simulink library "thc"  (R2021b)
settings: Solver=VariableStepAuto  StartTime=0.0  StopTime=10.0  RelTol=1e-3
undefined symbols (not defined in the file or in its folder): ATHC_APTCQA_X_C, ATHC_APTCQB_X_C, ATHC_dAy_X_C, ATHC_Qeq_X_kmh, ATHC_VbaseC_X_C, ATHC_VbaseC_Y_W, ATHC_VbaseD_X_C, ATHC_VbaseH_X_C, FALSE, KTHC_ACMaxMinT_sec, KTHC_aDeice_K, KTHC_AGSDefLv_K, KTHC_AGSLv1_K, KTHC_AGSLv2_K, KTHC_AGSLv3_K, KTHC_AGSLv4_K, KTHC_AGSLv5_K, KTHC_AirIntUpdateT_sec, KTHC_APTCOneZoneMax_W, KTHC_APTCPeriod_cnt, KTHC_APTCPWMEN_flg, KTHC_APTCQMaxC_W, KTHC_APTCQminC_W, KTHC_APTCQminD_W, KTHC_APTCQminRe1_W, KTHC_APTCQminRe_W, KTHC_APTCQoffT_cnt, KTHC_APTCQonT_cnt, KTHC_APTCRiLeMaxDff_W, KTHC_APTCRiLeMinDff_W, KTHC_BatInTempDef_C, KTHC_bDeice_K, KTHC_CompMaxDeice_rpm, KTHC_CompMinDeice_rpm, KTHC_CompSotxvOp_K, KTHC_CompSotxvOpLow_rpm, KTHC_CompSpdmax_rpm, KTHC_CompSpdmaxBC1_rpm, KTHC_CompSpdmaxBC_rpm, KTHC_CompSpdmid1_rpm, KTHC_CompSpdmid2_rpm, KTHC_CompSpdmid3_rpm, KTHC_CompSpdmid_rpm, KTHC_CompSpdmin_rpm, KTHC_DAPTCQ1_W, KTHC_DAPTCQ2_W, KTHC_DAPTCQ3_W, KTHC_DcChSetTemp_C, KTHC_DehumidityEN_flg, KTHC_DeiceCycTime_K, KTHC_DriveLevelWPTCBAH1_W, KTHC_DriveLevelWPTCBAH2_W, KTHC_DriveLevelWPTCBAH3_W, KTHC_DriveLevelWPTCBAH4_W, KTHC_DriveT1MinBAH_C, KTHC_DriveT2MaxBAH_C, KTHC_DriveT2MinBAH_C, KTHC_DriveT3MaxBAH_C, KTHC_DriveT3MinBAH_C, KTHC_DriveT4MaxBAH_C ... (+377)
libraries: simulink x145
(part 5 of 10)

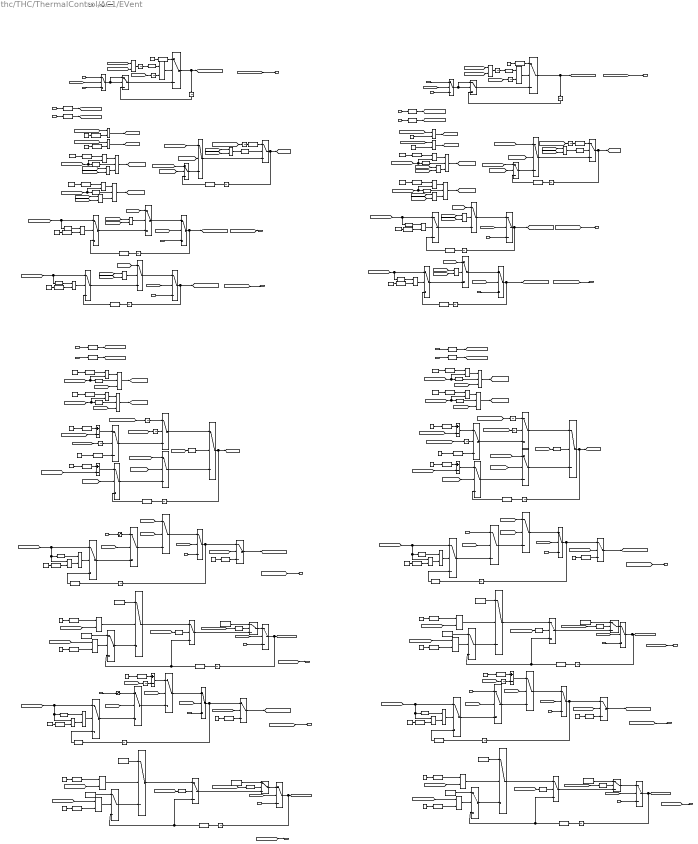
== system thc/THC/ThermalControl/AC1/EVent ==
  note: Driver Side
  note: Passenger Side
  fInitial : Inport
  VINP_IVIDrBlowerModeSta_enum : Inport  Port=2
  VINP_FDCTHCDrEVentModeStaM_enum : Inport  Port=3
  VINP_IVIPsBlowerModeSta_enum : Inport  Port=4
  VINP_FDCTHCPsEVentModeStaM_enum : Inport  Port=5
  VINP_IVIDrBlowerZSta_enum : Inport  Port=6
  VINP_IVICLBlowerZSta_enum : Inport  Port=7
  VINP_IVIPsBlowerZSta_enum : Inport  Port=8
  VINP_IVICRBlowerZSta_enum : Inport  Port=9
  VINP_FDCTHCDrEVentZStaM_enum : Inport  Port=10
  VINP_FDCTHCCLEVentZStaM_enum : Inport  Port=11
  VINP_FDCTHCPsEVentZStaM_enum : Inport  Port=12
  VINP_FDCTHCCREVentZStaM_enum : Inport  Port=13
  VINP_IVIDrBlowerYSta_enum : Inport  Port=14
  VINP_IVICLBlowerYSta_enum : Inport  Port=15
  VINP_ZFRTHCDrEVentActYSta_enum : Inport  Port=16
  VTHC_FDCTHCDrVentENM_flg : Inport  Port=17
  VINP_FDCTHCDrEVentYStaM_enum : Inport  Port=18
  VINP_ZFRTHCCLEVentActYSta_enum : Inport  Port=19
  VTHC_FDCTHCCLVentENM_flg : Inport  Port=20
  VINP_FDCTHCCLEVentYStaM_enum : Inport  Port=21
  VINP_IVIPsBlowerYSta_enum : Inport  Port=22
  VINP_IVICRBlowerYSta_enum : Inport  Port=23
  VINP_ZFRTHCPsEVentActYSta_enum : Inport  Port=24
  VTHC_FDCTHCPsVentENM_flg : Inport  Port=25
  VINP_FDCTHCPsEVentYStaM_enum : Inport  Port=26
  VINP_ZFRTHCCREVentActYSta_enum : Inport  Port=27
  VTHC_FDCTHCCRVentENM_flg : Inport  Port=28
  VINP_FDCTHCCREVentYStaM_enum : Inport  Port=29
  Add{,1..5} (6 alike) : Sum  Inputs=+-
  Constant{,1,4..5,7..8,10,14,18,23,25,28..29,33,38,40..42,45..46,48..51,53..54} (26 alike) : Constant  Value=100
  Constant11 : Constant  Value=3
  Constant12 : Constant  Value=50
  Constant{6,9,13,19,24,34,39,47} (8 alike) : Constant  Value=true
  Constant{15..16,20..21,30..31,35..36} (8 alike) : Constant  Value=126
  Constant{17,22,32,37} (4 alike) : Constant  Value=false
  Constant2 : Constant  Value=2
  Constant26 : Constant  Value=3
  Constant27 : Constant  Value=50
  Constant3 : Constant  Value=2
  Constant43 : Constant
  Constant44 : Constant
  Data Type Conversion{,1..20,22..25,27..35,37..40,42..65} (62 alike) : DataTypeConversion  OutDataTypeStr=uint8
  Data Type Conversion{21,26,36,41} (4 alike) : DataTypeConversion  OutDataTypeStr=boolean
  Detect Change{,1..17,19..20} (20 alike) : simulink/Logic and Bit Operations/Detect Change  vinit=0  OutDataTypeStr=boolean
  Detect Decrease : simulink/Logic and Bit Operations/Detect Decrease  vinit=0.0  OutDataTypeStr=boolean
  Detect Decrease1 : simulink/Logic and Bit Operations/Detect Decrease  vinit=0.0  OutDataTypeStr=boolean
  Detect Increase{,1..7} (8 alike) : simulink/Logic and Bit Operations/Detect Increase  vinit=0.0  OutDataTypeStr=boolean
  Logical Operator{,1..3,5..8} (8 alike) : Logic  Inputs=3  AllPortsSameDT=off  OutDataTypeStr=boolean
  Logical Operator{9..12,22..25} (8 alike) : Logic  AllPortsSameDT=off  OutDataTypeStr=boolean
  Logical Operator{4,13..21} (10 alike) : Logic  Operator=OR  AllPortsSameDT=off  OutDataTypeStr=boolean
  Relational Operator{,1,4..5,7..8,22..23} (8 alike) : RelationalOperator  OutDataTypeStr=boolean  RndMeth=Simplest
  Relational Operator{2,9..10,13,15..16,19,21,24..25,27..28} (12 alike) : RelationalOperator  Operator=<=  OutDataTypeStr=boolean  RndMeth=Simplest
  Relational Operator{3,6,11..12,14,17..18,20} (8 alike) : RelationalOperator  Operator===  OutDataTypeStr=boolean  RndMeth=Simplest
  Saturation : Saturate  UpperLimit=100  LowerLimit=0
  Saturation1 : Saturate  UpperLimit=100  LowerLimit=0
  Switch{,1..73} (74 alike) : Switch  Criteria=u2 > Threshold
  Unit Delay{,1..31} (32 alike) : UnitDelay  SampleTime=-1  HasFrameUpgradeWarning=on
  VTHC_FDCTHCDrEVentModeSta_enum : Outport
  VTHC_FDCTHCPsEVentModeSta_enum : Outport  Port=2
  VTHC_FDCTHCDrEVentZSta_enum : Outport  Port=3
  VTHC_FDCTHCCLEVentZSta_enum : Outport  Port=4
  VTHC_FDCTHCPsEVentZSta_enum : Outport  Port=5
  VTHC_FDCTHCCREVentZSta_enum : Outport  Port=6
  VTHC_FDCTHCDrEVentYSta_enum : Outport  Port=7
  VTHC_FDCTHCDrVentEN_flg : Outport  Port=8
  VTHC_FDCTHCCLEVentYSta_enum : Outport  Port=9
  VTHC_FDCTHCCLVentEN_flg : Outport  Port=10
  VTHC_FDCTHCPsEVentYSta_enum : Outport  Port=11
  VTHC_FDCTHCPsVentEN_flg : Outport  Port=12
  VTHC_FDCTHCCREVentYSta_enum : Outport  Port=13
  VTHC_FDCTHCCRVentEN_flg : Outport  Port=14
  wires:
  VINP_IVIPsBlowerYSta_enum/1 -> Data Type Conversion64/1
  Data Type Conversion65/1 -> [VINP_IVICRBlowerYSta_enum]
  VINP_IVICLBlowerYSta_enum/1 -> Data Type Conversion63/1
  VINP_IVIDrBlowerYSta_enum/1 -> Data Type Conversion62/1
  VINP_IVIPsBlowerZSta_enum/1 -> Data Type Conversion60/1
  VINP_IVICRBlowerZSta_enum/1 -> Data Type Conversion61/1
  VINP_IVICLBlowerZSta_enum/1 -> Data Type Conversion59/1
  Data Type Conversion56/1 -> [VINP_IVIDrBlowerZSta_enum]
  Unit Delay31/1 -> Switch45/1
  Unit Delay30/1 -> Add5/2
  Unit Delay29/1 -> Switch22/1
  Unit Delay28/1 -> Add4/2
  Relational Operator11/1 -> [DrBalanceMode]
  Logical Operator25/1 -> Switch38/2
  Constant53/1 -> Data Type Conversion57/1
  Data Type Conversion57/1 -> Relational Operator27/2
  Detect Change19/1 -> Logical Operator25/1
  [VINP_IVICLBlowerYSta_enum] -> Switch38/1, Relational Operator27/1, Detect Change19/1
  Relational Operator27/1 -> Logical Operator25/2
  Relational Operator24/1 -> Logical Operator24/2
  [VINP_IVIDrBlowerYSta_enum] -> Detect Change16/1, Relational Operator24/1, Switch29/1
  Detect Change16/1 -> Logical Operator24/1
  Data Type Conversion48/1 -> Relational Operator24/2
  Constant50/1 -> Data Type Conversion48/1
  Constant54/1 -> Data Type Conversion58/1
  Data Type Conversion58/1 -> Relational Operator28/2
  Detect Change20/1 -> Logical Operator23/1
  [VINP_IVIPsBlowerYSta_enum] -> Relational Operator28/1, Detect Change20/1, Switch52/1
  Relational Operator28/1 -> Logical Operator23/2
  Logical Operator23/1 -> Switch52/2
  Logical Operator22/1 -> Switch61/2
  Logical Operator24/1 -> Switch29/2
  Relational Operator25/1 -> Logical Operator22/2
  [VINP_IVICRBlowerYSta_enum] -> Detect Change17/1, Relational Operator25/1, Switch61/1
  Detect Change17/1 -> Logical Operator22/1
  Data Type Conversion55/1 -> Relational Operator25/2
  Constant51/1 -> Data Type Conversion55/1
  [VINP_IVICRBlowerZSta_enum] -> Detect Change15/1, Switch21/1
  Detect Change15/1 -> Relational Operator16/1
  Data Type Conversion47/1 -> Relational Operator16/2
  Constant49/1 -> Data Type Conversion47/1
  Relational Operator16/1 -> Switch21/2
  Relational Operator10/1 -> Switch18/2
  Constant48/1 -> Data Type Conversion31/1
  Data Type Conversion31/1 -> Relational Operator10/2
  Detect Change14/1 -> Relational Operator10/1
  [VINP_IVIPsBlowerZSta_enum] -> Detect Change14/1, Switch18/1
  [VINP_IVIDrBlowerZSta_enum] -> Detect Change13/1, Switch12/1
  Detect Change13/1 -> Relational Operator9/1
  Data Type Conversion15/1 -> Relational Operator9/2
  Constant42/1 -> Data Type Conversion15/1
  Relational Operator9/1 -> Switch12/2
  Relational Operator2/1 -> Switch15/2
  Constant28/1 -> Data Type Conversion8/1
  Data Type Conversion8/1 -> Relational Operator2/2
  Detect Change12/1 -> Relational Operator2/1
  [VINP_IVICLBlowerZSta_enum] -> Detect Change12/1, Switch15/1
  Switch73/1 -> Switch63/1
  [PsBalanceMode] -> Detect Increase6/1
  Detect Increase6/1 -> Switch73/2
  Constant13/1 -> Switch73/1
  Switch64/1 -> Switch73/3
  Switch72/1 -> Switch54/1
  Switch55/1 -> Switch72/3
  Constant9/1 -> Switch72/1
  Detect Increase7/1 -> Switch72/2
  [PsBalanceMode] -> Detect Increase7/1
  [VTHC_FDCTHCCRVentEN_flg] -> Unit Delay27/1
  Unit Delay26/1 -> Switch45/2
  Unit Delay25/1 -> Switch22/2
  [VTHC_FDCTHCDrVentEN_flg] -> Unit Delay25/1
  Unit Delay24/1 -> Switch26/2
  Saturation1/1 -> Switch28/1
  Saturation/1 -> Switch37/1
  Detect Increase2/1 -> Switch23/2
  [VTHC_FDCTHCDrEVentYSta_enum] -> Unit Delay29/1
  Switch71/1 -> Switch40/1
  Constant47/1 -> Switch71/1
  Detect Increase4/1 -> Switch71/2
  [DrBalanceMode] -> Detect Increase4/1
  [DrBalanceMode] -> Detect Increase5/1
  Detect Increase5/1 -> Switch70/2
  Constant6/1 -> Switch70/1
  Switch70/1 -> Switch31/1
  Logical Operator21/1 -> Detect Increase1/1
  [PsSweepMode] -> Logical Operator21/1
  [PsBalanceMode] -> Logical Operator21/2
  [PsSweepMode] -> Logical Operator20/1
  [PsBalanceMode] -> Logical Operator20/2
  [PsBalanceMode] -> Logical Operator19/2
  [PsSweepMode] -> Logical Operator19/1
  Logical Operator18/1 -> Logical Operator3/3
  [PsSweepMode] -> Logical Operator18/1
  [PsBalanceMode] -> Logical Operator18/2
  [PsBalanceMode] -> Logical Operator17/2
  [PsSweepMode] -> Logical Operator17/1
  Logical Operator17/1 -> Logical Operator2/3
  [DrBalanceMode] -> Logical Operator16/1
  [DrSweepMode] -> Logical Operator16/2
  [DrSweepMode] -> Logical Operator15/2
  [DrBalanceMode] -> Logical Operator15/1
  Logical Operator14/1 -> Detect Increase/1
  [DrSweepMode] -> Logical Operator14/2
  [DrBalanceMode] -> Logical Operator14/1
  [DrBalanceMode] -> Logical Operator13/1
  [DrSweepMode] -> Logical Operator13/2
  [DrSweepMode] -> Logical Operator4/2
  [DrBalanceMode] -> Logical Operator4/1
  Logical Operator4/1 -> Logical Operator/3
  [PsBalanceY] -> Unit Delay30/1
  Data Type Conversion54/1 -> Add5/1
  Constant46/1 -> Data Type Conversion54/1
  Add5/1 -> Switch59/1
  Add4/1 -> Switch36/1
  [DrBalanceY] -> Unit Delay28/1
  Data Type Conversion53/1 -> Add4/1
  Constant45/1 -> Data Type Conversion53/1
  Unit Delay23/1 -> Logical Operator11/2
  [PsBalanceMode] -> Unit Delay23/1
  Switch2/1 -> Switch69/3
  Switch69/1 -> [VTHC_FDCTHCPsEVentModeSta_enum], Unit Delay1/1
  [VTHC_FDCTHCCRVentEN_flg] -> Logical Operator12/2
  [VTHC_FDCTHCPsVentEN_flg] -> Logical Operator12/1
  Logical Operator12/1 -> Unit Delay22/1
  Unit Delay22/1 -> Detect Decrease1/1
  Detect Decrease1/1 -> Logical Operator11/1
  Logical Operator11/1 -> Switch69/2
  Data Type Conversion52/1 -> Switch69/1
  Constant44/1 -> Data Type Conversion52/1
  Switch/1 -> Switch68/3
  Constant43/1 -> Data Type Conversion51/1
  Data Type Conversion51/1 -> Switch68/1
  Logical Operator10/1 -> Switch68/2
  Unit Delay21/1 -> Logical Operator10/2
  [DrBalanceMode] -> Unit Delay21/1
  Data Type Conversion50/1 -> Relational Operator11/2
  Data Type Conversion49/1 -> Relational Operator6/2
  Detect Decrease/1 -> Logical Operator10/1
  Unit Delay20/1 -> Detect Decrease/1
  Logical Operator9/1 -> Unit Delay20/1
  [VTHC_FDCTHCDrVentEN_flg] -> Logical Operator9/1
  [VTHC_FDCTHCCLVentEN_flg] -> Logical Operator9/2
  [DrBalanceMode] -> Logical Operator6/3
  Constant29/1 -> Data Type Conversion34/1
  VINP_FDCTHCDrEVentYStaM_enum/1 -> Switch35/3
  Unit Delay8/1 -> Data Type Conversion14/1
  Data Type Conversion10/1 -> Switch12/3
  Switch31/1 -> Unit Delay12/1, [VTHC_FDCTHCDrVentEN_flg]
  Constant37/1 -> Switch65/1
  [fInitial] -> Switch1/2
  Constant22/1 -> Switch42/1
  Data Type Conversion2/1 -> Relational Operator4/1
  [VTHC_FDCTHCPsEVentZSta_enum] -> VTHC_FDCTHCPsEVentZSta_enum/1
  VINP_ZFRTHCCREVentActYSta_enum/1 -> Switch60/1
  Switch68/1 -> [VTHC_FDCTHCDrEVentModeSta_enum], Unit Delay/1
  Data Type Conversion44/1 -> Relational Operator21/2
  Data Type Conversion39/1 -> Relational Operator19/2
  Relational Operator5/1 -> Logical Operator3/1
  [VINP_IVICLBlowerYSta_enum] -> Add1/2
  Relational Operator8/1 -> Logical Operator6/1
  Data Type Conversion64/1 -> [VINP_IVIPsBlowerYSta_enum]
  Switch23/1 -> Unit Delay8/1, [DrBalanceY]
  Data Type Conversion63/1 -> [VINP_IVICLBlowerYSta_enum]
  Data Type Conversion/1 -> Relational Operator/1
  [fInitial] -> Switch40/2
  VINP_IVIDrBlowerZSta_enum/1 -> Data Type Conversion56/1
  Data Type Conversion12/1 -> Switch18/3
  [VINP_IVICLBlowerYSta_enum] -> Relational Operator14/2
  Data Type Conversion36/1 -> Switch57/3, Switch55/3
  Switch7/1 -> Switch8/3
  Data Type Conversion22/1 -> Switch30/3
  Constant16/1 -> Data Type Conversion22/1
  [VTHC_FDCTHCPsVentEN_flg] -> VTHC_FDCTHCPsVentEN_flg/1
  Detect Change1/1 -> Logical Operator1/2
  [DrBalanceMode] -> Logical Operator5/3
  Data Type Conversion29/1 -> Relational Operator15/2
  [VINP_IVIPsBlowerYSta_enum] -> Detect Change10/1
  [VINP_IVICLBlowerZSta_enum] -> Switch4/1
  Relational Operator12/1 -> Switch33/2
  [DrBalanceMode] -> Switch27/2
  [VINP_IVICRBlowerYSta_enum] -> Detect Change11/1
  [DrYupdate] -> Switch24/2
  [PsBalanceZ] -> Switch19/1
  [fInitial] -> Switch31/2
  Switch34/1 -> Switch33/3
  Switch49/1 -> Switch45/3
  Constant10/1 -> Data Type Conversion18/1
  Unit Delay/1 -> Switch/3
  Switch56/1 -> Switch55/1
  Switch66/1 -> Switch65/3
  [VINP_IVIDrBlowerYSta_enum] -> Relational Operator12/2
  Data Type Conversion14/1 -> Switch25/3
  Unit Delay16/1 -> Data Type Conversion36/1
  [PsBalanceZ] -> Switch16/1
  VINP_FDCTHCDrEVentZStaM_enum/1 -> Switch11/3
  Constant21/1 -> Data Type Conversion27/1
  [VTHC_FDCTHCPsEVentYSta_enum] -> VTHC_FDCTHCPsEVentYSta_enum/1
  Switch61/1 -> Switch60/3
  Constant15/1 -> Data Type Conversion23/1
  Unit Delay11/1 -> Data Type Conversion20/1
  Data Type Conversion59/1 -> [VINP_IVICLBlowerZSta_enum]
  Constant24/1 -> Switch43/1
  Switch42/1 -> Switch41/1
  Switch51/1 -> Switch50/3
  Relational Operator15/1 -> Switch43/2
  Unit Delay19/1 -> Data Type Conversion30/1
  Add1/1 -> Switch25/1
  [VTHC_FDCTHCCLVentEN_flg] -> VTHC_FDCTHCCLVentEN_flg/1
  [PsBalanceMode] -> Switch50/2
  [VINP_IVICRBlowerYSta_enum] -> Relational Operator20/2
  Data Type Conversion38/1 -> Relational Operator18/1
  Data Type Conversion46/1 -> Relational Operator23/1
  Constant38/1 -> Data Type Conversion44/1
  Switch65/1 -> Switch64/1
  Relational Operator20/1 -> Switch65/2
  Constant35/1 -> Data Type Conversion43/1
  Data Type Conversion43/1 -> Relational Operator20/1
  [fInitial] -> Switch58/2
  [PsZupdate] -> Switch8/2
  Detect Change7/1 -> Switch41/2
  Add/1 -> Switch26/1
  [VTHC_FDCTHCPsEVentYSta_enum] -> Unit Delay31/1
  Switch30/1 -> [VTHC_FDCTHCDrEVentYSta_enum]
  Switch58/1 -> Unit Delay15/1, Switch53/1
  Detect Change8/1 -> Logical Operator7/2
  [DrZupdate] -> Switch5/2
  Detect Increase/1 -> Switch6/2
  Unit Delay10/1 -> Data Type Conversion17/1
  [VINP_IVICRBlowerZSta_enum] -> Switch7/1
  [VTHC_FDCTHCDrEVentModeSta_enum] -> VTHC_FDCTHCDrEVentModeSta_enum/1
  Constant40/1 -> Data Type Conversion45/1
  Constant41/1 -> Data Type Conversion46/1
  Switch20/1 -> [VTHC_FDCTHCCREVentZSta_enum], Unit Delay7/1
  Relational Operator22/1 -> Logical Operator7/1
  [fInitial] -> Switch67/2
  [VINP_IVIPsBlowerYSta_enum] -> Relational Operator19/1
  Switch53/1 -> [VTHC_FDCTHCPsEVentYSta_enum]
  [VINP_IVIPsBlowerZSta_enum] -> Switch8/1
  [VINP_IVIPsBlowerYSta_enum] -> Relational Operator22/2, Detect Change8/1
  Relational Operator19/1 -> Switch57/2
  Add2/1 -> Switch49/1
  Detect Change11/1 -> Switch64/2
  Data Type Conversion7/1 -> Relational Operator8/1
  Switch59/1 -> Switch67/1
  Data Type Conversion35/1 -> Switch52/3
  Switch11/1 -> [VTHC_FDCTHCDrEVentZSta_enum], Unit Delay4/1
  Switch47/1 -> Switch46/3
  Switch3/1 -> Switch2/1, Switch2/2
  Constant12/1 -> Data Type Conversion16/1
  Logical Operator7/1 -> [PsYupdate]
  Switch45/1 -> Switch46/1
  [PsSweepMode] -> Switch51/2
  Switch41/1 -> Switch71/3
  [PsBalanceMode] -> Detect Increase3/1
  [VTHC_FDCTHCPsVentEN_flg] -> Switch53/2
  [VTHC_FDCTHCDrEVentModeSta_enum] -> Relational Operator6/1
  Constant2/1 -> Data Type Conversion49/1
  [VTHC_FDCTHCCLEVentYSta_enum] -> VTHC_FDCTHCCLEVentYSta_enum/1
  [VTHC_FDCTHCCLVentEN_flg] -> Switch39/2
  Relational Operator3/1 -> [PsSweepMode]
  Constant3/1 -> Relational Operator3/2
  [VTHC_FDCTHCPsEVentModeSta_enum] -> Relational Operator3/1
  Data Type Conversion27/1 -> Switch39/3
  Data Type Conversion20/1 -> Switch29/3
  Switch16/1 -> Switch17/1
  [VINP_IVIDrBlowerYSta_enum] -> Relational Operator7/2, Detect Change4/1
  Switch17/1 -> Unit Delay6/1, [VTHC_FDCTHCPsEVentZSta_enum]
  [fInitial] -> Switch17/2
  Detect Change4/1 -> Logical Operator5/2
  VINP_FDCTHCPsEVentZStaM_enum/1 -> Switch17/3
  Logical Operator19/1 -> Switch16/2
  [VINP_IVICRBlowerYSta_enum] -> Relational Operator21/1
  [VINP_IVIDrBlowerYSta_enum] -> Switch24/1
  Relational Operator1/1 -> Logical Operator1/1
  Unit Delay2/1 -> Data Type Conversion4/1
  Switch25/1 -> Switch24/3
  [fInitial] -> Switch14/2
  [VINP_IVICLBlowerYSta_enum] -> Relational Operator15/1
  Data Type Conversion24/1 -> Relational Operator13/2
  [VTHC_FDCTHCDrEVentModeSta_enum] -> Relational Operator11/1
  Switch27/1 -> Switch35/1
  [VTHC_FDCTHCCLEVentZSta_enum] -> VTHC_FDCTHCCLEVentZSta_enum/1
  VTHC_FDCTHCDrVentENM_flg/1 -> Switch31/3
  [fInitial] -> Switch3/2
  Switch1/1 -> Switch/2, Switch/1
  VINP_IVIDrBlowerModeSta_enum/1 -> Switch1/1
  Relational Operator13/1 -> Switch34/2
  Constant11/1 -> Data Type Conversion50/1
  [VTHC_FDCTHCPsEVentModeSta_enum] -> VTHC_FDCTHCPsEVentModeSta_enum/1
  Logical Operator8/1 -> [CRYupdate]
  VINP_IVIPsBlowerModeSta_enum/1 -> Switch3/1
  Unit Delay14/1 -> Data Type Conversion26/1
  [DrBalanceZ] -> Switch10/1
  Data Type Conversion42/1 -> Switch62/3
  [VTHC_FDCTHCDrEVentZSta_enum] -> Unit Delay10/1
  Data Type Conversion17/1 -> Switch6/1
  Logical Operator1/1 -> [CLZupdate]
  [VINP_IVIDrBlowerZSta_enum] -> Detect Change/1, Relational Operator/2
  Switch32/1 -> Switch70/3
  [VINP_IVICRBlowerZSta_enum] -> Detect Change3/1, Relational Operator5/2
  Constant25/1 -> Data Type Conversion33/1
  [PsYupdate] -> Switch47/2
  Switch50/1 -> Switch58/1
  [fInitial] -> Switch54/2
  Data Type Conversion28/1 -> Relational Operator14/1
  [VTHC_FDCTHCCREVentYSta_enum] -> Add2/2
  Detect Change6/1 -> Switch32/2
  [PsBalanceMode] -> Logical Operator7/3
  Add3/1 -> Switch48/1
  [VTHC_FDCTHCCRVentEN_flg] -> VTHC_FDCTHCCRVentEN_flg/1
  [VINP_IVIPsBlowerYSta_enum] -> Switch47/1
  Switch46/1 -> Unit Delay19/1, [PsBalanceY]
  Switch62/1 -> [VTHC_FDCTHCCREVentYSta_enum]
  Detect Change9/1 -> Logical Operator8/2
  Data Type Conversion34/1 -> Add3/1
  [VTHC_FDCTHCCLVentEN_flg] -> Unit Delay24/1
  Unit Delay9/1 -> Data Type Conversion9/1
  Detect Increase3/1 -> Switch46/2
  Constant17/1 -> Switch33/1
  Data Type Conversion16/1 -> Switch26/3
  Unit Delay5/1 -> Data Type Conversion11/1
  [CLYupdate] -> Switch25/2
  [VTHC_FDCTHCDrEVentZSta_enum] -> VTHC_FDCTHCDrEVentZSta_enum/1
  Relational Operator/1 -> Logical Operator/1
  [VTHC_FDCTHCPsEVentZSta_enum] -> Unit Delay9/1
  Switch26/1 -> Switch22/3
  Data Type Conversion18/1 -> Add/1
  Switch4/1 -> Switch5/3
  Data Type Conversion60/1 -> [VINP_IVIPsBlowerZSta_enum]
  Logical Operator/1 -> [DrZupdate]
  Constant18/1 -> Data Type Conversion24/1
  Switch29/1 -> Switch28/3
  Unit Delay4/1 -> Data Type Conversion10/1
  Constant20/1 -> Data Type Conversion28/1
  VINP_FDCTHCDrEVentModeStaM_enum/1 -> Switch1/3
  Relational Operator6/1 -> [DrSweepMode]
  VINP_ZFRTHCDrEVentActYSta_enum/1 -> Saturation1/1
  [fInitial] -> Switch11/2
  Switch21/1 -> Switch19/3
  Logical Operator20/1 -> Switch19/2
  Switch19/1 -> Switch20/1
  [PsBalanceMode] -> Logical Operator8/3
  [fInitial] -> Switch20/2
  VINP_FDCTHCCREVentZStaM_enum/1 -> Switch20/3
  [VINP_IVICLBlowerYSta_enum] -> Detect Change7/1
  Switch18/1 -> Switch16/3
  Unit Delay7/1 -> Data Type Conversion13/1
  [VINP_IVICRBlowerYSta_enum] -> Add3/2
  Unit Delay6/1 -> Data Type Conversion12/1
  Relational Operator17/1 -> [PsBalanceMode]
  Switch14/1 -> Unit Delay5/1, [VTHC_FDCTHCCLEVentZSta_enum]
  Unit Delay18/1 -> Data Type Conversion41/1
  [CLZupdate] -> Switch4/2
  Data Type Conversion26/1 -> Switch41/3, Switch43/3
  Detect Change/1 -> Logical Operator/2
  Constant/1 -> Data Type Conversion/1
  Switch5/1 -> Switch6/3
  [VINP_IVIDrBlowerYSta_enum] -> Detect Change6/1
  [VINP_IVIDrBlowerZSta_enum] -> Switch5/1
  Constant34/1 -> Switch57/1
  VINP_ZFRTHCCLEVentActYSta_enum/1 -> Saturation/1
  Constant1/1 -> Data Type Conversion1/1
  Data Type Conversion1/1 -> Relational Operator1/1
  [VINP_IVICLBlowerYSta_enum] -> Detect Change5/1, Relational Operator8/2
  [VINP_IVICLBlowerZSta_enum] -> Relational Operator1/2, Detect Change1/1
  Detect Change2/1 -> Logical Operator2/2
  fInitial/1 -> [fInitial]
  VINP_FDCTHCPsEVentModeStaM_enum/1 -> Switch3/3
  Unit Delay1/1 -> Switch2/3
  VTHC_FDCTHCPsVentENM_flg/1 -> Switch54/3
  VINP_ZFRTHCPsEVentActYSta_enum/1 -> Switch51/1
  Data Type Conversion40/1 -> Switch61/3
  Switch60/1 -> Switch59/3
  [PsSweepMode] -> Switch60/2
  Data Type Conversion6/1 -> Relational Operator7/1
  Data Type Conversion33/1 -> Add2/1
  Constant33/1 -> Data Type Conversion39/1
  Switch54/1 -> [VTHC_FDCTHCPsVentEN_flg], Unit Delay16/1
  [PsBalanceMode] -> Switch59/2
  Detect Change10/1 -> Switch55/2
  Data Type Conversion13/1 -> Switch21/3
  [PsBalanceY] -> Switch50/1
  Constant36/1 -> Data Type Conversion42/1
  Constant30/1 -> Data Type Conversion38/1
  [VINP_IVIPsBlowerYSta_enum] -> Relational Operator18/2
  [VTHC_FDCTHCCRVentEN_flg] -> Switch62/2
  Relational Operator21/1 -> Switch66/2
  Data Type Conversion37/1 -> Switch53/3
  [VTHC_FDCTHCCREVentYSta_enum] -> VTHC_FDCTHCCREVentYSta_enum/1
  Switch57/1 -> Switch56/3
  Unit Delay15/1 -> Data Type Conversion35/1
  Data Type Conversion30/1 -> Switch48/3
  Constant31/1 -> Data Type Conversion37/1
  Switch67/1 -> Switch62/1, Unit Delay17/1
  Switch52/1 -> Switch51/3
  Unit Delay17/1 -> Data Type Conversion40/1
  Unit Delay27/1 -> Switch49/2
  Constant32/1 -> Switch56/1
  Data Type Conversion32/1 -> Switch49/3
  Constant27/1 -> Data Type Conversion32/1
  [CRYupdate] -> Switch48/2
  Switch6/1 -> Unit Delay2/1, [DrBalanceZ]
  Data Type Conversion4/1 -> Switch4/3
  Unit Delay13/1 -> Data Type Conversion25/1
  Switch63/1 -> [VTHC_FDCTHCCRVentEN_flg], Unit Delay18/1
  Switch39/1 -> [VTHC_FDCTHCCLEVentYSta_enum]
  Data Type Conversion25/1 -> Switch38/3
  Switch44/1 -> Switch39/1, Unit Delay13/1
  Switch37/1 -> Switch36/3
  Switch38/1 -> Switch37/3
  [DrSweepMode] -> Switch37/2
  [DrBalanceMode] -> Switch36/2
  Data Type Conversion5/1 -> Switch7/3
  [DrBalanceY] -> Switch27/1
  VTHC_FDCTHCCLVentENM_flg/1 -> Switch40/3
  Switch40/1 -> [VTHC_FDCTHCCLVentEN_flg], Unit Delay14/1
  [VTHC_FDCTHCCREVentZSta_enum] -> VTHC_FDCTHCCREVentZSta_enum/1
  Logical Operator13/1 -> Logical Operator1/3
  Switch22/1 -> Switch23/1
  Switch36/1 -> Switch44/1
  Switch48/1 -> Switch47/3
  Logical Operator5/1 -> [DrYupdate]
  Unit Delay12/1 -> Data Type Conversion21/1
  VINP_IVICRBlowerYSta_enum/1 -> Data Type Conversion65/1
  Data Type Conversion9/1 -> Switch9/1
  Switch24/1 -> Switch23/3
  [DrSweepMode] -> Switch28/2
  Data Type Conversion11/1 -> Switch15/3
  Constant7/1 -> Data Type Conversion6/1
  [VINP_IVIPsBlowerZSta_enum] -> Relational Operator4/2, Detect Change2/1
  Data Type Conversion61/1 -> [VINP_IVICRBlowerZSta_enum]
  Unit Delay3/1 -> Data Type Conversion5/1
  Switch9/1 -> [PsBalanceZ], Unit Delay3/1
  Detect Increase1/1 -> Switch9/2
  [CRZupdate] -> Switch7/2
  Logical Operator2/1 -> [PsZupdate]
  Switch8/1 -> Switch9/3
  Logical Operator3/1 -> [CRZupdate]
  Detect Change3/1 -> Logical Operator3/2
  Switch28/1 -> Switch27/3
  Constant4/1 -> Data Type Conversion2/1
  Data Type Conversion3/1 -> Relational Operator5/1
  Constant5/1 -> Data Type Conversion3/1
  Data Type Conversion62/1 -> [VINP_IVIDrBlowerYSta_enum]
  Relational Operator4/1 -> Logical Operator2/1
  Relational Operator18/1 -> Switch56/2
  Switch10/1 -> Switch11/1
  Switch13/1 -> Switch14/1
  Switch15/1 -> Switch13/3
  VINP_FDCTHCCLEVentZStaM_enum/1 -> Switch14/3
  Logical Operator16/1 -> Switch13/2
  Constant19/1 -> Switch34/1
  Switch12/1 -> Switch10/3
  [DrBalanceMode] -> Detect Increase2/1
  [DrBalanceZ] -> Switch13/1
  [VTHC_FDCTHCDrVentEN_flg] -> Switch30/2
  VTHC_FDCTHCCRVentENM_flg/1 -> Switch63/3
  Data Type Conversion41/1 -> Switch64/3, Switch66/3
  Constant8/1 -> Data Type Conversion7/1
  [VTHC_FDCTHCPsEVentModeSta_enum] -> Relational Operator17/1
  Constant26/1 -> Relational Operator17/2
  [fInitial] -> Switch63/2
  Data Type Conversion23/1 -> Relational Operator12/1
  [VTHC_FDCTHCDrEVentYSta_enum] -> VTHC_FDCTHCDrEVentYSta_enum/1
  Logical Operator15/1 -> Switch10/2
  Constant23/1 -> Data Type Conversion29/1
  Switch43/1 -> Switch42/3
  Relational Operator14/1 -> Switch42/2
  [VTHC_FDCTHCDrVentEN_flg] -> VTHC_FDCTHCDrVentEN_flg/1
  [fInitial] -> Switch35/2
  Switch33/1 -> Switch32/1
  Switch35/1 -> Unit Delay11/1, Switch30/1
  VINP_FDCTHCCLEVentYStaM_enum/1 -> Switch44/3
  Data Type Conversion21/1 -> Switch34/3, Switch32/3
  Logical Operator6/1 -> [CLYupdate]
  Detect Change5/1 -> Logical Operator6/2
  Relational Operator7/1 -> Logical Operator5/1
  Data Type Conversion45/1 -> Relational Operator22/1
  [VTHC_FDCTHCPsVentEN_flg] -> Unit Delay26/1
  Relational Operator23/1 -> Logical Operator8/1
  [VINP_IVICRBlowerYSta_enum] -> Detect Change9/1, Relational Operator23/2
  VINP_FDCTHCCREVentYStaM_enum/1 -> Switch67/3
  Constant39/1 -> Switch66/1
  VINP_FDCTHCPsEVentYStaM_enum/1 -> Switch58/3
  [fInitial] -> Switch44/2
  [VINP_IVIDrBlowerYSta_enum] -> Relational Operator13/1
  Data Type Conversion19/1 -> Add1/1
  Constant14/1 -> Data Type Conversion19/1
  [VTHC_FDCTHCCLEVentYSta_enum] -> Add/2

== system thc/THC/ThermalControl/AC1/ModMath2 ==
  Dividend : Inport
  Divisor : Inport  Port=2
  Abs : Abs
  Constant : Constant  Value=eps
  Data Type Conversion : DataTypeConversion
  Data Type Conversion1 : DataTypeConversion
  Data Type Conversion2 : DataTypeConversion  OutDataTypeStr=single
  Divide : Product  Inputs=*/
  Equal : RelationalOperator  Operator=<=  OutDataTypeStr=boolean  RndMeth=Simplest
  Floor : Rounding
  Minus : Sum  Inputs=+-
  Product : Product
  Switch : Switch  Criteria=u2 > Threshold
  Remainder : Outport
  wires:
  [Divisor] -> Abs/1
  Product/1 -> Data Type Conversion/1
  Divide/1 -> Data Type Conversion2/1
  [Divisor] -> Product/2
  Abs/1 -> Equal/1
  [Divisor] -> Divide/2
  Data Type Conversion1/1 -> Product/1
  Floor/1 -> Data Type Conversion1/1
  Dividend/1 -> [Dividend]
  [Dividend] -> Minus/1
  Data Type Conversion/1 -> Minus/2
  Data Type Conversion2/1 -> Floor/1
  Minus/1 -> Switch/3
  [Dividend] -> Switch/1
  Switch/1 -> Remainder/1
  [Dividend] -> Divide/1
  Constant/1 -> Equal/2
  Equal/1 -> Switch/2
  Divisor/1 -> [Divisor]

== system thc/THC/ThermalControl/AC1/Subsystem ==
  IVI_FGSAirInt_Cmd : Inport
  FGSAirIntStaM : Inport  Port=2
  IVI_FGSCh_Cmd : Inport  Port=3
  FGSChStaM : Inport  Port=4
  PwrSta : Inport  Port=5
  IVI_IONSW_Cmd : Inport  Port=6
  "IONSWStaM " : Inport  Port=7
  FGS_MotorInit_Sta : Inport  Port=8
  FGS_AirInt_Sta : Inport  Port=9
  Chart : Stateflow chart  TreatAsAtomicUnit=on
  Constant : Constant  Value=3
  Constant{1,3..4,9} (4 alike) : Constant
  Constant10 : Constant  Value=3
  Constant{2,6..8} (4 alike) : Constant  Value=0
  Constant5 : Constant  Value=3
  Data Type Conversion : DataTypeConversion
  Detect Increase : simulink/Logic and Bit Operations/Detect Increase  vinit=0.0  OutDataTypeStr=boolean
  Logical Operator : Logic  Operator=NOT  AllPortsSameDT=off  OutDataTypeStr=boolean
  Logical Operator1 : Logic  AllPortsSameDT=off  OutDataTypeStr=boolean
  Logical Operator2 : Logic  AllPortsSameDT=off  OutDataTypeStr=boolean
  Relational Operator : RelationalOperator  Operator=<=  OutDataTypeStr=boolean  RndMeth=Simplest
  Relational Operator{1..4} (4 alike) : RelationalOperator  Operator=>  OutDataTypeStr=boolean  RndMeth=Simplest
  Switch{,1..8} (9 alike) : Switch  Criteria=u2 > Threshold
  Unit Delay{,1..5} (6 alike) : UnitDelay  SampleTime=-1  HasFrameUpgradeWarning=on
  FGSAirIntSta : Outport
  FGSChSta : Outport  Port=2
  FGSAirIntCmd : Outport  Port=3
  FGSFuncSta : Outport  Port=4
  FGSChCmd : Outport  Port=5
  FDC_FGS_IONSW_Sta : Outport  Port=6
  FDC_FGS_ION_Cmd : Outport  Port=7
  FGSLearn : Outport  Port=8
  wires:
  Relational Operator1/1 -> Switch2/2
  Switch2/1 -> Switch3/1
  Constant8/1 -> Switch6/3
  FGSAirIntStaM/1 -> Switch1/3
  [PwrSta] -> Chart/2(PwrSta)
  Chart/2(FGSEnable) -> [FGSEnable]
  Switch8/1 -> Switch7/1
  Switch4/1 -> Switch3/3
  Unit Delay4/1 -> Switch7/2
  IVI_FGSAirInt_Cmd/1 -> Switch/1, Relational Operator/1
  Chart/1(FGSLearn) -> FGSLearn/1
  Constant7/1 -> Relational Operator3/2
  [PwrSta] -> Relational Operator4/1
  Unit Delay5/1 -> Switch8/3, Logical Operator/1
  Switch7/1 -> Unit Delay5/1, Logical Operator1/1, FDC_FGS_IONSW_Sta/1
  Constant4/1 -> Switch4/3
  FGS_MotorInit_Sta/1 -> Chart/1(FGS_MotorInit_Sta)
  Switch3/1 -> Switch6/1, FGSChSta/1, Unit Delay3/1
  FGS_AirInt_Sta/1 -> Chart/4(FGS_AirInt_Sta)
  Relational Operator3/1 -> Data Type Conversion/1
  Detect Increase/1 -> Switch8/2
  Unit Delay2/1 -> Switch3/2
  [FGSEnable] -> Logical Operator2/2
  PwrSta/1 -> [PwrSta], Relational Operator2/1
  [PwrON] -> Switch5/2
  [IVI_FGSCh_Cmd] -> Chart/3(IVI_FGSCh_Cmd)
  Unit Delay/1 -> Switch1/2
  Switch/1 -> Switch1/1
  Constant10/1 -> Relational Operator4/2
  Logical Operator2/1 -> [PwrON]
  Switch6/1 -> FGSChCmd/1
  Switch5/1 -> Relational Operator3/1, FGSAirIntCmd/1
  Unit Delay1/1 -> Switch/3
  "IONSWStaM "/1 -> Switch7/3
  [PwrON] -> Switch6/2
  Constant6/1 -> Switch5/3
  Constant5/1 -> Relational Operator2/2
  Data Type Conversion/1 -> FGSFuncSta/1
  Relational Operator2/1 -> Logical Operator2/1
  Constant3/1 -> Unit Delay2/1
  Unit Delay3/1 -> Switch2/3
  Constant1/1 -> Unit Delay/1
  FGSChStaM/1 -> Switch4/2, Switch4/1
  IVI_IONSW_Cmd/1 -> Detect Increase/1
  Relational Operator4/1 -> Logical Operator1/2
  Constant2/1 -> Relational Operator1/2
  Relational Operator/1 -> Switch/2
  IVI_FGSCh_Cmd/1 -> [IVI_FGSCh_Cmd]
  Logical Operator/1 -> Switch8/1
  Switch1/1 -> FGSAirIntSta/1, Switch5/1, Unit Delay1/1
  [IVI_FGSCh_Cmd] -> Relational Operator1/1, Switch2/1
  Constant9/1 -> Unit Delay4/1
  Constant/1 -> Relational Operator/2
  Logical Operator1/1 -> FDC_FGS_ION_Cmd/1

== system thc/THC/ThermalControl/THCM_Conctrl/AGSandFan ==
  AGSLV : Inport
  Fan_Err : Inport  Port=2
  FAN : Inport  Port=3
  Compare To Constant : simulink/Logic and Bit Operations/Compare To Constant  relop=>  const=1  OutDataTypeStr=boolean
  Constant : Constant  Value=KTHC_AGSLv1_K
  Constant1 : Constant  Value=KTHC_AGSLv2_K
  Constant2 : Constant  Value=KTHC_AGSLv3_K
  Constant3 : Constant  Value=KTHC_AGSLv4_K
  Constant4 : Constant  Value=KTHC_AGSLv5_K
  Constant5 : Constant  Value=0
  Constant6 : Constant  Value=KTHC_AGSDefLv_K
  Constant7 : Constant  Value=KTHC_ErrHandleEN_flg
  Logical Operator : Logic  Inputs=3  AllPortsSameDT=off  OutDataTypeStr=boolean
  Multiport Switch : MultiPortSwitch  Inputs=6  DiagnosticForDefault=None
  Switch : Switch  Criteria=u2 > Threshold
  AGSOut : Outport
  wires:
  Constant7/1 -> Logical Operator/3
  Constant6/1 -> Switch/1
  Switch/1 -> AGSOut/1
  Logical Operator/1 -> Switch/2
  Multiport Switch/1 -> Switch/3
  Compare To Constant/1 -> Logical Operator/2
  Fan_Err/1 -> Logical Operator/1
  FAN/1 -> Compare To Constant/1
  AGSLV/1 -> Multiport Switch/1
  Constant5/1 -> Multiport Switch/7
  Constant4/1 -> Multiport Switch/6
  Constant3/1 -> Multiport Switch/5
  Constant/1 -> Multiport Switch/2
  Constant1/1 -> Multiport Switch/3
  Constant2/1 -> Multiport Switch/4

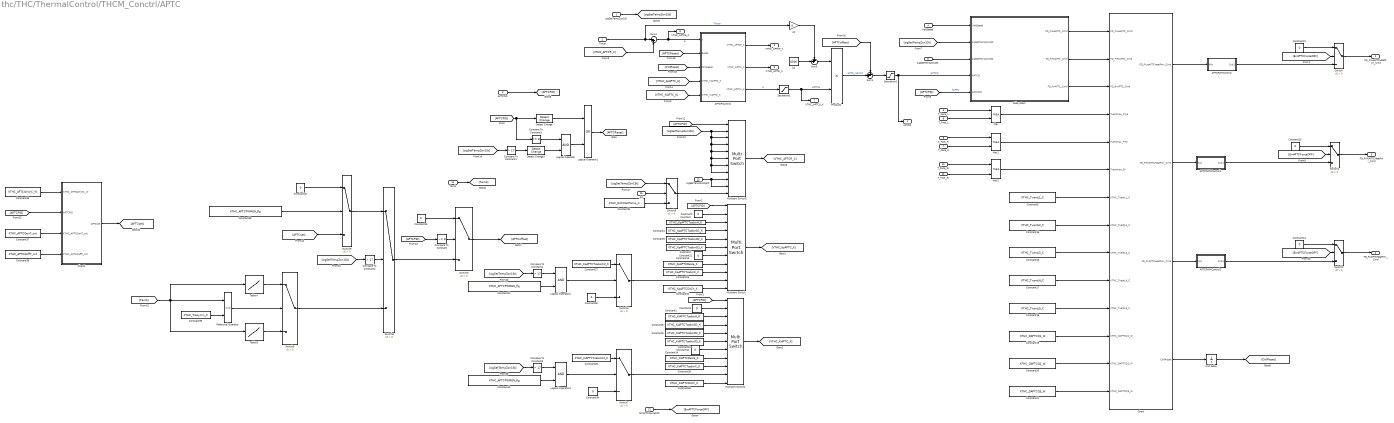
== system thc/THC/ThermalControl/THCM_Conctrl/APTC ==
  sigSetTempZon1St : Inport
  Tincar : Inport  Port=2
  APTCPID : Inport  Port=3
  VehSpeed : Inport  Port=4
  sigSetTempZon2St : Inport  Port=5
  T_Face_L : Inport  Port=6
  T_Face_R : Inport  Port=7
  T_Foot_L : Inport  Port=8
  T_Foot_R : Inport  Port=9
  T_Face_Rr : Inport  Port=10
  T_Foot_Rr : Inport  Port=11
  ErrAPTCForceOFF : Inport  Port=12
  sigSetTempZon1StC : Inport  Port=13
  Tamb : Inport  Port=14
  AC : Inport  Port=15
  APTCPIControl : Subsystem
  APTCPWMControl : Subsystem
  APTCPWMControl1 : Subsystem
  APTCPWMControl2 : Subsystem
  Chart : Stateflow chart  TreatAsAtomicUnit=on
  Chart1 : Stateflow chart  TreatAsAtomicUnit=on
  Compare To Constant : simulink/Logic and Bit Operations/Compare To Constant  relop=~=  const=8  OutDataTypeStr=boolean
  Compare To Constant{1..2,4,6} (4 alike) : simulink/Logic and Bit Operations/Compare To Constant  relop=>  const=17  OutDataTypeStr=boolean
  Compare To Constant3 : simulink/Logic and Bit Operations/Compare To Constant  relop===  const=8  OutDataTypeStr=boolean
  Constant : Constant  Value=KTHC_KpAPTCTcabinH_K
  Constant1 : Constant  Value=KTHC_KiAPTCTcabinH_K
  Constant10 : Constant  Value=KTHC_KiAPTCTcabinD3_K
  Constant{2..3,11..12,22..24,29..30,34,40} (11 alike) : Constant  Value=0
  Constant13 : Constant  Value=KTHC_KpAPTCDeice_K
  Constant14 : Constant  Value=KTHC_KiAPTCDeice_K
  Constant15 : Constant  Value=KTHC_TventL2_C
  Constant16 : Constant  Value=KTHC_TventL3_C
  Constant17 : Constant  Value=KTHC_TventL4_C
  Constant18 : Constant  Value=KTHC_TventL5_C
  Constant19 : Constant  Value=KTHC_DAPTCQ1_W
  Constant20 : Constant  Value=KTHC_DAPTCQ2_W
  Constant21 : Constant  Value=KTHC_DAPTCQ3_W
  Constant25 : Constant  Value=KTHC_KpAPTCTcabinC_K
  Constant26 : Constant  Value=KTHC_KiAPTCTcabinC_K
  Constant27 : Constant  Value=KTHC_KpAPTCTcabinC2_K
  Constant28 : Constant  Value=KTHC_KiAPTCTcabinC2_K
  Constant31 : Constant  Value=KTHC_DcChSetTemp_C
  Constant32 : Constant  Value=KTHC_KpAPTCDcCh_K
  Constant33 : Constant  Value=KTHC_KiAPTCDcCh_K
  Constant35 : Constant  Value=KTHC_Trecymin_C
  Constant36 : Constant  Value=KTHC_APTCQminC_W
  Constant37 : Constant  Value=KTHC_APTCQonT_cnt
  Constant38 : Constant  Value=KTHC_APTCQoffT_cnt
  Constant39 : Constant  Value=KTHC_APTCPWMEN_flg
  Constant4 : Constant  Value=KTHC_KpAPTCTcabinD1_K
  Constant41 : Constant  Value=KTHC_APTCPWMEN_flg
  Constant42 : Constant  Value=KTHC_APTCPWMEN_flg
  Constant5 : Constant  Value=KTHC_TventL1_C
  Constant6 : Constant  Value=KTHC_KpAPTCTcabinD2_K
  Constant7 : Constant  Value=KTHC_KpAPTCTcabinD3_K
  Constant8 : Constant  Value=KTHC_KiAPTCTcabinD1_K
  Constant9 : Constant  Value=KTHC_KiAPTCTcabinD2_K
  Detect Change : simulink/Logic and Bit Operations/Detect Change  vinit=0  OutDataTypeStr=boolean
  Detect Change1 : simulink/Logic and Bit Operations/Detect Change  vinit=0  OutDataTypeStr=boolean
  Logical Operator : Logic  AllPortsSameDT=off  OutDataTypeStr=boolean
  Logical Operator1 : Logic  Operator=OR  AllPortsSameDT=off  OutDataTypeStr=boolean
  Logical Operator2 : Logic  AllPortsSameDT=off  OutDataTypeStr=boolean
  Logical Operator3 : Logic  AllPortsSameDT=off  OutDataTypeStr=boolean
  Max : MinMax  Function=max  Inputs=2
  Max1 : MinMax  Function=max  Inputs=2
  Max2 : MinMax  Function=max  Inputs=2
  Multiport Switch : MultiPortSwitch  DataPortOrder=Zero-based contiguous  Inputs=10  zeroidx=on
  Multiport Switch1 : MultiPortSwitch  DataPortOrder=Zero-based contiguous  Inputs=10  zeroidx=on
  Multiport Switch2 : MultiPortSwitch  DataPortOrder=Zero-based contiguous  Inputs=10  zeroidx=on
  Product1 : Product
  Relational Operator : RelationalOperator  OutDataTypeStr=boolean  RndMeth=Simplest
  Saturation1 : Saturate  UpperLimit=1  LowerLimit=0
  Saturation2 : Saturate  UpperLimit=6500  LowerLimit=0
  Subsystem : Subsystem
  Sum1 : Sum  Inputs=++|
  Sum3 : Sum  Inputs=|-+
  Sum5 : Sum  Inputs=++|
  Switch{,1..9} (10 alike) : Switch  Criteria=u2 > Threshold
  Table A : Lookup_n-D  NumberOfTableDimensions=1  BreakpointsForDimension1=ATHC_APTCQA_X_C  Table=MTHC_APTCQA_Y_W  InternalRulePriority=Speed  RndMeth=Simplest  InputSameDT=on
  Table B : Lookup_n-D  NumberOfTableDimensions=1  BreakpointsForDimension1=ATHC_APTCQB_X_C  Table=MTHC_APTCQB_Y_W  InternalRulePriority=Speed  RndMeth=Simplest  InputSameDT=on
  Unit Delay : UnitDelay  SampleTime=-1  HasFrameUpgradeWarning=on
  a1 : Gain  Gain=0
  b1 : Constant  Value=6500
  APTCQ : Outport
  FD_FrLeAPTCHeatPwr_Cmd : Outport  Port=2
  FD_FrRiAPTCHeatPwr_Cmd : Outport  Port=3
  FD_RrAPTCHeatPwr_Cmd : Outport  Port=4
  VTHC_APTCP_K : Outport  Port=5
  VTHC_APTCI_K : Outport  Port=6
  VTHC_APTCU_K : Outport  Port=7
  VTHC_APTCe_K : Outport  Port=8
  wires:
  [CtrlReset] -> APTCPIControl/3(CtrlReset)
  Unit Delay/1 -> [CtrlReset]
  Chart/4(CtrlReset) -> Unit Delay/1
  Constant33/1 -> Multiport Switch1/11
  Constant32/1 -> Multiport Switch/11
  Switch6/1 -> Multiport Switch2/11
  Constant31/1 -> Switch6/3
  [sigSetTempZon1St] -> Switch6/1
  AC/1 -> Switch6/2
  [APTCoffset] -> Sum1/1
  Sum1/1 -> Saturation2/1
  Switch3/1 -> [APTCoffset]
  Table B/1 -> Switch5/3
  Table A/1 -> Switch5/1
  Relational Operator/1 -> Switch5/2
  [Tamb] -> Table A/1, Table B/1, Relational Operator/1
  Tamb/1 -> [Tamb]
  Constant29/1 -> Switch3/1
  Compare To Constant1/1 -> Detect Change1/1
  [sigSetTempZon1St] -> Compare To Constant1/1
  [APTCPID] -> Compare To Constant/1
  sigSetTempZon1StC/1 -> Multiport Switch2/9, Multiport Switch2/10
  Constant26/1 -> Multiport Switch1/9
  Constant25/1 -> Multiport Switch/9
  [sigSetTempZon1St] -> Multiport Switch2/2, Multiport Switch2/3, Multiport Switch2/4, Multiport Switch2/5, Multiport Switch2/6, Multiport Switch2/7, Multiport Switch2/8
  [APTCPID] -> Multiport Switch2/1
  Multiport Switch2/1 -> [VTHC_APTCR_C]
  Switch2/1 -> FD_RrAPTCHeatPwr_Cmd/1
  Constant24/1 -> Switch2/1
  [ErrAPTCForceOFF] -> Switch2/2
  APTCPWMControl2/1(Out1) -> Switch2/3
  Switch1/1 -> FD_FrRiAPTCHeatPwr_Cmd/1
  [ErrAPTCForceOFF] -> Switch1/2
  Constant23/1 -> Switch1/1
  Constant22/1 -> Switch/1
  [ErrAPTCForceOFF] -> Switch/2
  Switch/1 -> FD_FrLeAPTCHeatPwr_Cmd/1
  ErrAPTCForceOFF/1 -> [ErrAPTCForceOFF]
  APTCPWMControl/1(Out1) -> Switch/3
  Constant21/1 -> Chart/14(KTHC_DAPTCQ3_W)
  Constant20/1 -> Chart/13(KTHC_DAPTCQ2_W)
  Constant19/1 -> Chart/12(KTHC_DAPTCQ1_W)
  Constant18/1 -> Chart/11(KTHC_TventL5_C)
  Constant17/1 -> Chart/10(KTHC_TventL4_C)
  Constant16/1 -> Chart/9(KTHC_TventL3_C)
  Constant15/1 -> Chart/8(KTHC_TventL2_C)
  Constant5/1 -> Chart/7(KTHC_TventL1_C)
  Max2/1 -> Chart/6(Tventmax_Rr)
  Max1/1 -> Chart/5(Tventmax_FrRi)
  Subsystem/3(FD_RrAPTC_Cmd) -> Chart/3(FD_RrAPTC_Cmd)
  Subsystem/2(FD_FrRiAPTC_Cmd) -> Chart/2(FD_FrRiAPTC_Cmd)
  Subsystem/1(FD_FrLeAPTC_Cmd) -> Chart/1(FD_FrLeAPTC_Cmd)
  Max/1 -> Chart/4(Tventmax_FrLe)
  T_Foot_Rr/1 -> Max2/2
  T_Face_R/1 -> Max1/2
  T_Foot_R/1 -> Max1/1
  T_Face_L/1 -> Max/1
  T_Foot_L/1 -> Max/2
  T_Face_Rr/1 -> Max2/1
  Constant14/1 -> Multiport Switch1/8
  Constant13/1 -> Multiport Switch/8
  [APTCPID] -> Subsystem/5(APTCPID)  "fAPTC"
  sigSetTempZon1St/1 -> [sigSetTempZon1St]
  [sigSetTempZon1St] -> Subsystem/2(sigSetTempZon1St)
  sigSetTempZon2St/1 -> Subsystem/3(sigSetTempZon2St)
  VehSpeed/1 -> Subsystem/1(VehSpeed)
  Constant12/1 -> Multiport Switch1/7
  Constant11/1 -> Multiport Switch/7
  [VTHC_KiAPTC_K] -> APTCPIControl/5(VTHC_KiAPTC_K)
  [VTHC_KpAPTC_K] -> APTCPIControl/4(VTHC_KpAPTC_K)
  Constant10/1 -> Multiport Switch1/6
  Constant9/1 -> Multiport Switch1/5
  Constant8/1 -> Multiport Switch1/4
  Constant7/1 -> Multiport Switch/6
  Constant6/1 -> Multiport Switch/5
  Constant4/1 -> Multiport Switch/4
  [APTCPID] -> Multiport Switch1/1
  Constant3/1 -> Multiport Switch1/2
  Multiport Switch1/1 -> [VTHC_KiAPTC_K]
  Multiport Switch/1 -> [VTHC_KpAPTC_K]
  Constant2/1 -> Multiport Switch/2
  [APTCPID] -> Multiport Switch/1
  APTCPIControl/2(VTHC_APTCI_K) -> VTHC_APTCI_K/1
  APTCPIControl/1(VTHC_APTCP_K) -> VTHC_APTCP_K/1
  Constant1/1 -> Multiport Switch1/3
  Constant/1 -> Multiport Switch/3
  Saturation2/1 -> Subsystem/4(APTCQ), APTCQ/1  "APTCQ"
  [APTCReset] -> APTCPIControl/2(Reset)
  APTCPIControl/3(VTHC_APTCU_K) -> Saturation1/1  "U"
  Sum3/1 -> APTCPIControl/1(x), VTHC_APTCe_K/1  "e"
  b1/1 -> Sum5/2
  Sum5/1 -> Product1/1
  Tincar/1 -> Sum3/1, a1/1  "Tincar"
  Saturation1/1 -> Product1/2, VTHC_APTCU_K/1  "APTC%"
  Product1/1 -> Sum1/2  "APTC_nolimit"
  a1/1 -> Sum5/1
  [VTHC_APTCR_C] -> Sum3/2
  Chart/1(FD_FrLeAPTCHeatPwr_Cmd) -> APTCPWMControl/1(Win)
  Chart/2(FD_FrRiAPTCHeatPwr_Cmd) -> APTCPWMControl1/1(Win)
  APTCPWMControl1/1(Out1) -> Switch1/3
  Chart/3(FD_RrAPTCHeatPwr_Cmd) -> APTCPWMControl2/1(Win)
  Switch5/1 -> Switch8/3
  Detect Change/1 -> Logical Operator1/1
  Compare To Constant3/1 -> Logical Operator/1
  Detect Change1/1 -> Logical Operator/2
  Logical Operator/1 -> Logical Operator1/2
  Logical Operator1/1 -> [APTCReset]
  [APTCPID] -> Compare To Constant3/1, Detect Change/1
  APTCPID/1 -> [APTCPID]
  Switch4/1 -> Multiport Switch/10
  Switch7/1 -> Multiport Switch1/10
  [sigSetTempZon1St] -> Compare To Constant4/1
  Logical Operator2/1 -> Switch4/2
  Constant28/1 -> Switch7/1
  Constant27/1 -> Switch4/1
  Constant30/1 -> Switch4/3
  Constant34/1 -> Switch7/3
  Constant35/1 -> Relational Operator/2
  [sigSetTempZon1St] -> Compare To Constant2/1
  Compare To Constant/1 -> Switch3/2
  Constant37/1 -> Chart1/3(KTHC_APTCQonT_cnt)
  [APTCPID] -> Chart1/2(APTCPID)
  Constant36/1 -> Chart1/1(KTHC_APTCQminC_W)
  Chart1/1(APTCset) -> [APTCset]
  Constant38/1 -> Chart1/4(KTHC_APTCQoffT_cnt)
  Switch8/1 -> Switch3/3
  Compare To Constant2/1 -> Switch8/2
  Switch9/1 -> Switch8/1
  Constant39/1 -> Switch9/2
  Constant40/1 -> Switch9/1
  [APTCset] -> Switch9/3
  Compare To Constant4/1 -> Logical Operator2/1
  Constant41/1 -> Logical Operator2/2
  Constant42/1 -> Logical Operator3/2
  Compare To Constant6/1 -> Logical Operator3/1
  [sigSetTempZon1St] -> Compare To Constant6/1
  Logical Operator3/1 -> Switch7/2
